simulink model "hihi"  (Simulink 8.6)
settings: Solver=VariableStepAuto  StartTime=0.0  StopTime=inf  RelTol=1e-3
libraries: simulink x4
settings Model: Creator=user  LastModifiedBy=achal
settings DataIOCC: SaveFormat=Dataset  SignalLoggingSaveFormat=Dataset
settings OptimizationCC: ExpressionDepthLimit=128
settings DebuggingCC: UnderspecifiedInitializationDetection=Simplified  MergeDetectMultiDrivingBlocksExec=error  SolverPrmCheckMsg=none  FcnCallInpInsideContextMsg=EnableAllAsError  StateNameClashWarn=none
settings HardwareCC: ProdBitPerPointer=64  ProdLargestAtomicFloat=Float  ProdIntDivRoundTo=Zero  ProdEndianess=LittleEndian  ProdWordSize=64  ProdHWDeviceType=Intel->x86-64 (Windows64)
settings GRTTargetCC: GeneratePreprocessorConditionals=Use local settings  CombineOutputUpdateFcns=on  GRTInterface=off
settings ConfigComp: CovModelRefEnable=off
settings ConfigurationSet: Description=SimMechanics 2G

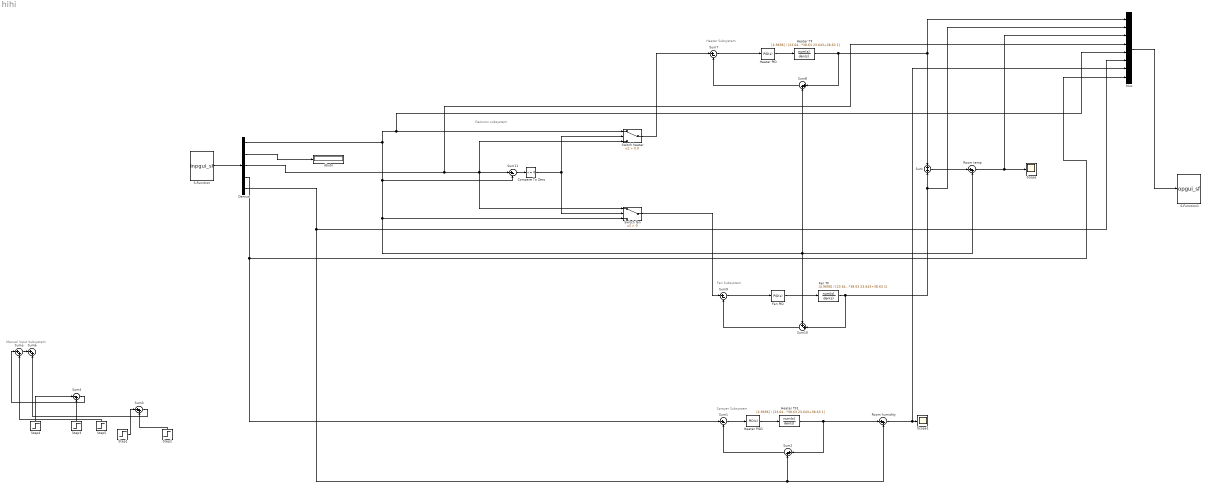
== system hihi ==
  note: Sprayer Subsystem
  note: Manual Input Subsystem
  note: Fan Subsystem
  note: Heater Subsystem
  note: Decision subsystem
  Compare To Zero : simulink/Logic and Bit Operations/Compare To Zero  relop=<=  OutDataTypeStr=boolean
  Demux : Demux  Outputs=5
  Fan PID : simulink/Continuous/PID Controller  Controller=PID  TimeDomain=Continuous-time  SampleTime=-1  IntegratorMethod=Forward Euler  FilterMethod=Forward Euler  Form=Parallel  UseFilter=on  ControllerParametersSource=internal  P=2.07829396686203  I=0.0344337981619069  D=31.1730262957423  N=19.3761241130532  InitialConditionSource=internal  InitialConditionForIntegrator=0  InitialConditionForFilter=0  ExternalReset=none  LimitOutput=off  UpperSaturationLimit=inf  LowerSaturationLimit=-inf  LinearizeAsGain=on  AntiWindupMode=none  Kb=1  TrackingMode=off  Kt=1  PParamMin=[]  PParamMax=[]  IParamMin=[]  IParamMax=[]  DParamMin=[]  DParamMax=[]  NParamMin=[]  NParamMax=[]  KbParamMin=[]  KbParamMax=[]  KtParamMin=[]  KtParamMax=[]  POutMin=[]  POutMax=[]  IOutMin=[]  IOutMax=[]  DOutMin=[]  DOutMax=[]  NOutMin=[]  NOutMax=[]  KbOutMin=[]  KbOutMax=[]  KtOutMin=[]  KtOutMax=[]  IntegratorOutMin=[]  IntegratorOutMax=[]  FilterOutMin=[]  FilterOutMax=[]  SumOutMin=[]  SumOutMax=[]  SumI1OutMin=[]  SumI1OutMax=[]  SumI2OutMin=[]  SumI2OutMax=[]  SumI3OutMin=[]  SumI3OutMax=[]  SumDOutMin=[]  SumDOutMax=[]  SaturationOutMin=[]  SaturationOutMax=[]  IntegratorContinuousStateAttributes=''  IntegratorStateMustResolveToSignalObject=off  IntegratorRTWStateStorageClass=Auto  FilterContinuousStateAttributes=''  FilterStateMustResolveToSignalObject=off  FilterRTWStateStorageClass=Auto  DifferentiatorICPrevScaledInput=0  DifferentiatorOutMin=[]  DifferentiatorOutMax=[]
  Fan TF : TransferFcn  Numerator=[4.9696]  Denominator=[23.643*38.63 23.643+38.63 1]
  Heater PID : simulink/Continuous/PID Controller  Controller=PID  TimeDomain=Continuous-time  SampleTime=-1  IntegratorMethod=Forward Euler  FilterMethod=Forward Euler  Form=Parallel  UseFilter=on  ControllerParametersSource=internal  P=2.07829396686203  I=0.0344337981619069  D=31.1730262957423  N=19.3761241130532  InitialConditionSource=internal  InitialConditionForIntegrator=0  InitialConditionForFilter=0  ExternalReset=none  LimitOutput=off  UpperSaturationLimit=inf  LowerSaturationLimit=-inf  LinearizeAsGain=on  AntiWindupMode=none  Kb=1  TrackingMode=off  Kt=1  PParamMin=[]  PParamMax=[]  IParamMin=[]  IParamMax=[]  DParamMin=[]  DParamMax=[]  NParamMin=[]  NParamMax=[]  KbParamMin=[]  KbParamMax=[]  KtParamMin=[]  KtParamMax=[]  POutMin=[]  POutMax=[]  IOutMin=[]  IOutMax=[]  DOutMin=[]  DOutMax=[]  NOutMin=[]  NOutMax=[]  KbOutMin=[]  KbOutMax=[]  KtOutMin=[]  KtOutMax=[]  IntegratorOutMin=[]  IntegratorOutMax=[]  FilterOutMin=[]  FilterOutMax=[]  SumOutMin=[]  SumOutMax=[]  SumI1OutMin=[]  SumI1OutMax=[]  SumI2OutMin=[]  SumI2OutMax=[]  SumI3OutMin=[]  SumI3OutMax=[]  SumDOutMin=[]  SumDOutMax=[]  SaturationOutMin=[]  SaturationOutMax=[]  IntegratorContinuousStateAttributes=''  IntegratorStateMustResolveToSignalObject=off  IntegratorRTWStateStorageClass=Auto  FilterContinuousStateAttributes=''  FilterStateMustResolveToSignalObject=off  FilterRTWStateStorageClass=Auto  DifferentiatorICPrevScaledInput=0  DifferentiatorOutMin=[]  DifferentiatorOutMax=[]
  Heater PID1 : simulink/Continuous/PID Controller  Controller=PID  TimeDomain=Continuous-time  SampleTime=-1  IntegratorMethod=Forward Euler  FilterMethod=Forward Euler  Form=Parallel  UseFilter=on  ControllerParametersSource=internal  P=2.07829396686203  I=0.0344337981619069  D=31.1730262957423  N=19.3761241130532  InitialConditionSource=internal  InitialConditionForIntegrator=0  InitialConditionForFilter=0  ExternalReset=none  LimitOutput=off  UpperSaturationLimit=inf  LowerSaturationLimit=-inf  LinearizeAsGain=on  AntiWindupMode=none  Kb=1  TrackingMode=off  Kt=1  PParamMin=[]  PParamMax=[]  IParamMin=[]  IParamMax=[]  DParamMin=[]  DParamMax=[]  NParamMin=[]  NParamMax=[]  KbParamMin=[]  KbParamMax=[]  KtParamMin=[]  KtParamMax=[]  POutMin=[]  POutMax=[]  IOutMin=[]  IOutMax=[]  DOutMin=[]  DOutMax=[]  NOutMin=[]  NOutMax=[]  KbOutMin=[]  KbOutMax=[]  KtOutMin=[]  KtOutMax=[]  IntegratorOutMin=[]  IntegratorOutMax=[]  FilterOutMin=[]  FilterOutMax=[]  SumOutMin=[]  SumOutMax=[]  SumI1OutMin=[]  SumI1OutMax=[]  SumI2OutMin=[]  SumI2OutMax=[]  SumI3OutMin=[]  SumI3OutMax=[]  SumDOutMin=[]  SumDOutMax=[]  SaturationOutMin=[]  SaturationOutMax=[]  IntegratorContinuousStateAttributes=''  IntegratorStateMustResolveToSignalObject=off  IntegratorRTWStateStorageClass=Auto  FilterContinuousStateAttributes=''  FilterStateMustResolveToSignalObject=off  FilterRTWStateStorageClass=Auto  DifferentiatorICPrevScaledInput=0  DifferentiatorOutMin=[]  DifferentiatorOutMax=[]
  Heater TF : TransferFcn  Numerator=[4.9696]  Denominator=[23.643*38.63 23.643+38.63 1]
  Heater TF1 : TransferFcn  Numerator=[4.9696]  Denominator=[23.643*38.63 23.643+38.63 1]
  Mux : Mux  Inputs=8
  Room humidity : Sum  Inputs=|++
  Room temp : Sum  Inputs=|++
  S-Function : S-Function  FunctionName=inpgui_sf  Parameters=0  SFunctionDeploymentMode=off  EnableBusSupport=off
  S-Function1 : S-Function  FunctionName=opgui_sf  Parameters=0.005  SFunctionDeploymentMode=off  EnableBusSupport=off
  Scope : Scope
  Scope1 : Scope
  Step1 : Step  Time=40  SampleTime=0
  Step2 : Step  Time=60  SampleTime=0
  Step3 : Step  Time=80  After=3  SampleTime=0
  Step4 : Step  Time=140  After=8  SampleTime=0
  Step5 : Step  Time=240  SampleTime=0
  Sum : Sum  Inputs=+|+
  Sum{1,7,9,11} (4 alike) : Sum  Inputs=|+-
  Sum10 : Sum  Inputs=++|
  Sum{2..3,5..6,8} (5 alike) : Sum  Inputs=|++
  Sum4 : Sum  Inputs=|-+
  Switch fan : Switch  Criteria=u2 > Threshold
  Switch heater : Switch  Criteria=u2 > Threshold  Threshold=0.0
  dbutn : Display
  wires:
  S-Function/1 -> Demux/1
  Demux/2 -> dbutn/1
  Mux/1 -> S-Function1/1
  Sum/1 -> Room temp/1
  Room temp/1 -> Mux/3, Scope/1
  Heater TF/1 -> Mux/1, Sum/1, Sum8/1
  Fan TF/1 -> Mux/2, Sum/2, Sum10/2
  Sum11/1 -> Compare To Zero/1
  Demux/3 -> Mux/4, Sum11/1, Switch fan/1, Switch heater/3
  Compare To Zero/1 -> Switch heater/2, Switch fan/2
  Switch heater/1 -> Sum7/1
  Sum8/1 -> Sum7/2
  Heater PID/1 -> Heater TF/1
  Sum7/1 -> Heater PID/1
  Demux/1 -> Sum11/2, Switch fan/3, Room temp/2, Sum10/1, Sum8/2, Mux/5, Switch heater/1
  Fan PID/1 -> Fan TF/1
  Sum9/1 -> Fan PID/1
  Sum10/1 -> Sum9/2
  Switch fan/1 -> Sum9/1
  Step3/1 -> Sum4/2
  Sum3/1 -> Sum6/2
  Step4/1 -> Sum4/1
  Step1/1 -> Sum3/1
  Sum4/1 -> Sum5/1
  Step2/1 -> Sum3/2
  Step5/1 -> Sum5/2
  Sum5/1 -> Sum6/1
  Room humidity/1 -> Mux/7, Scope1/1
  Heater TF1/1 -> Room humidity/1, Sum2/1
  Heater PID1/1 -> Heater TF1/1
  Sum1/1 -> Heater PID1/1
  Sum2/1 -> Sum1/2
  Demux/4 -> Mux/8, Sum1/1
  Demux/5 -> Mux/6, Sum2/2, Room humidity/2
